simulink library "Library_Octocopter"  (R2015b)
settings: Solver=VariableStepAuto  StartTime=0.0  StopTime=10.0  RelTol=1e-3
values from neighbouring files (symbols this model uses):
  AoAMax = 18    [MainDataFile.m]
  ChordBlade = 0.2    [MainDataFile.m]
  DiameterBlade = 8    [MainDataFile.m]
  MassBlade = 35    [MainDataFile.m]
  RPMMax = 6400    [MainDataFile.m]
  s = saveObjectImpl@matlab.System(obj)    [moving_average.m]
  ThicknessBlade = 0.04    [MainDataFile.m]
  TransmissionRatio = 12    [MainDataFile.m]
undefined symbols (not defined in the file or in its folder): X, Y, Z
libraries: sm_lib x10, nesl_utility x9
settings Model: Creator=John  LastModifiedBy=hielke

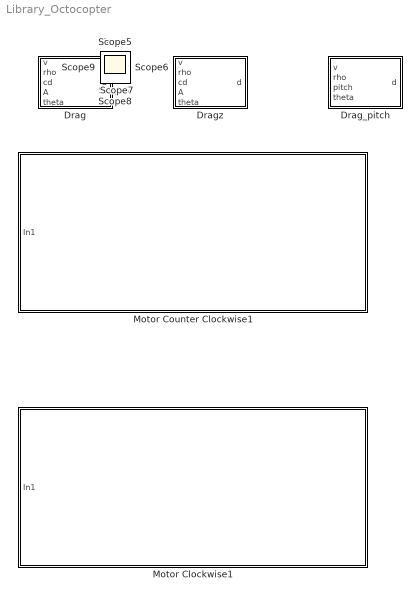
== system Library_Octocopter ==
  Drag : MATLAB Function  TreatAsAtomicUnit=on  SystemSampleTime=1
      settings: MinAlgLoopOccurrences=on  RTWSystemCode=Inline
  Drag_pitch : MATLAB Function  TreatAsAtomicUnit=on  SystemSampleTime=1
      settings: MinAlgLoopOccurrences=on  RTWSystemCode=Inline
  "Dragz " : MATLAB Function  TreatAsAtomicUnit=on  SystemSampleTime=1
      settings: MinAlgLoopOccurrences=on  RTWSystemCode=Inline
  Motor Clockwise1 : Subsystem
  Motor Counter Clockwise1 : Subsystem
  Scope{,1..9} (10 alike) : Scope

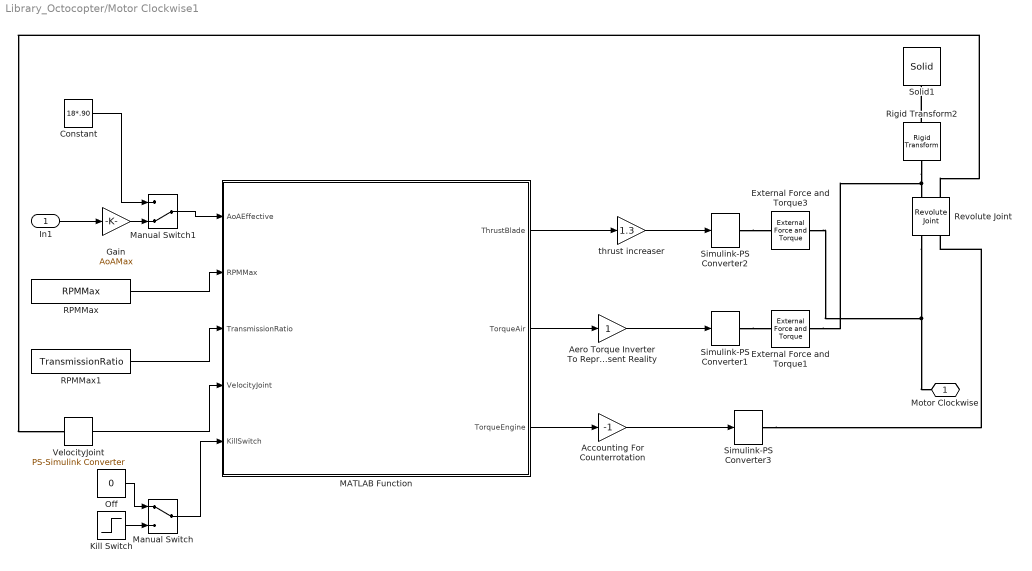
== system Library_Octocopter/Motor Clockwise1 ==
  In1 : Inport
  Accounting For Counterrotation : Gain  Gain=-1
  Aero Torque Inverter To Represent Reality : Gain
  Constant : Constant  Value=18*.90
  External Force and Torque1 : sm_lib/Forces and Torques/External Force and Torque  ForceResolutionFrame=AttachedFrame  EnableForceX=off  EnableForceY=off  EnableForceZ=off  EnableForce=off  TorqueResolutionFrame=AttachedFrame  EnableTorqueX=off  EnableTorqueY=off  EnableTorqueZ=on  EnableTorque=off  BlockFunction=simmechanics.library.forces_torques.external_force_torque
  External Force and Torque3 : sm_lib/Forces and Torques/External Force and Torque  ForceResolutionFrame=AttachedFrame  EnableForceX=off  EnableForceY=off  EnableForceZ=on  EnableForce=off  TorqueResolutionFrame=AttachedFrame  EnableTorqueX=off  EnableTorqueY=off  EnableTorqueZ=off  EnableTorque=off  BlockFunction=simmechanics.library.forces_torques.external_force_torque
  Gain : Gain  Gain=AoAMax
  Kill Switch : Step  Time=10
  MATLAB Function : MATLAB Function  TreatAsAtomicUnit=on
  Manual Switch : ManualSwitch
  Manual Switch1 : ManualSwitch  CurrentSetting=0
  Off : Constant  Value=0
  RPMMax : Constant  Value=RPMMax
  RPMMax1 : Constant  Value=TransmissionRatio
  Revolute Joint : sm_lib/Joints/Revolute Joint  SenseConstraintForce=off  SenseConstraintForceX=off  SenseConstraintForceY=off  SenseConstraintForceZ=off  SenseConstraintTorque=off  SenseConstraintTorqueX=off  SenseConstraintTorqueY=off  SenseConstraintTorqueZ=off  SenseTotalForce=off  SenseTotalForceX=off  SenseTotalForceY=off  SenseTotalForceZ=off  SenseTotalTorque=off  SenseTotalTorqueX=off  SenseTotalTorqueY=off  SenseTotalTorqueZ=off  CompositeWrenchDir=FollowerOnBase  CompositeWrenchFrame=BaseFrame  EquilibriumPosition=0  EquilibriumPositionUnits=deg  SpringStiffness=0  SpringStiffnessUnits=N*m/deg  DampingCoefficient=0  DampingCoefficientUnits=N*m/(deg/s)  TorqueActuationMode=InputTorque  MotionActuationMode=ComputedMotion  SensePosition=off  SenseVelocity=on  SenseAcceleration=off  SenseTorqueForce=off  PositionTargetSpecify=off  PositionTargetPriority=High  PositionTargetValue=0  PositionTargetValueUnits=deg  VelocityTargetSpecify=off  VelocityTargetPriority=High  VelocityTargetValue=0  VelocityTargetValueUnits=deg/s  BlockFunction=simmechanics.library.joints.revolute_joint
  Rigid Transform2 : sm_lib/Frames and Transforms/Rigid Transform  TranslationMethod=None  TranslationLengthUnit=m  TranslationStandardAxis=+Z  TranslationStandardOffset=0  TranslationCartesianOffset=[0 0 0]  TranslationROffset=0  TranslationROffsetUnits=m  TranslationZOffset=0  TranslationZOffsetUnits=m  TranslationThetaOffset=0  TranslationThetaOffsetUnits=deg  RotationMethod=StandardAxis  RotationAngleUnits=deg  RotationStandardAxis=+X  RotationAngle=90  RotationArbitraryAxis=[0 0 1]  FollAlignAxisA=+X  BaseAlignAxisA=+Y  FollAlignAxisB=+Y  BaseAlignAxisB=+Z  RotationSequenceAxes=FollowerAxes  RotationSequence=XYX  RotationSequenceAngles=[0 0 0]  RotationSequenceAnglesUnits=deg  RotationMatrix=[1 0 0; 0 1 0; 0 0 1]  BlockFunction=simmechanics.library.frames_transforms.rigid_transform
  Simulink-PS Converter1 : nesl_utility/Simulink-PS Converter  PhysicalDomain=network_engine_domain  SubClassName=ps_input  LeftPortType=input  RightPortType=output  PseudoPeriodic=off  Frequencies=[]  NoiseDistribution=none  NoiseParameters=[]  Unit=1  AffineConversion=off  InputFiltering=off  SimscapeFilterOrder=1  InputFilterTimeConstant=0.001  UdotUserProvided=1
  Simulink-PS Converter2 : nesl_utility/Simulink-PS Converter  PhysicalDomain=network_engine_domain  SubClassName=ps_input  LeftPortType=input  RightPortType=output  PseudoPeriodic=off  Frequencies=[]  NoiseDistribution=none  NoiseParameters=[]  Unit=1  AffineConversion=off  InputFiltering=off  SimscapeFilterOrder=1  InputFilterTimeConstant=0.001  UdotUserProvided=1
  Simulink-PS Converter3 : nesl_utility/Simulink-PS Converter  PhysicalDomain=network_engine_domain  SubClassName=ps_input  LeftPortType=input  RightPortType=output  PseudoPeriodic=off  Frequencies=[]  NoiseDistribution=none  NoiseParameters=[]  Unit=1  AffineConversion=off  InputFiltering=off  SimscapeFilterOrder=1  InputFilterTimeConstant=0.001  UdotUserProvided=1
  Solid1 : sm_lib/Body Elements/Solid  InertiaType=CalculateFromGeometry  Mass=MassBlade  MassUnits=kg  CenterOfMass=[0 0 0]  CenterOfMassUnits=m  MomentsOfInertia=[1 1 1]  MomentsOfInertiaUnits=kg*m^2  ProductsOfInertia=[0 0 0]  ProductsOfInertiaUnits=kg*m^2  DensityBased=off  Density=DensityBlade  DensityUnits=kg/(m^3)  DoExposeReferenceFrame=on  SerializedFrames=<Frames/>  GraphicType=FromGeometry  MarkerShape=Sphere  MarkerSize=10  MarkerSizeUnits=m  GraphicVisPropType=SimpleVisualProperties  GraphicDiffuseColor=[0.5 0.5 0.5]  GraphicSpecularColor=[0.5 0.5 0.5 1.0]  GraphicAmbientColor=[0.15 0.15 0.15 1.0]  GraphicEmissiveColor=[0.0 0.0 0.0 1.0]  GraphicShininess=75  GraphicOpacity=1.0  GeometryShape=Ellipsoid  RectangleSize=[1 1]  RectangleSizeUnits=m  BrickDimensions=[1 1 1]  BrickDimensionUnits=m  CylinderRadius=1  CylinderRadiusUnits=m  CylinderLength=1  CylinderLengthUnits=m  SphereRadius=1  SphereRadiusUnits=m  EllipsoidRadii=[DiameterBlade/2 ThicknessBlade/2 ChordBlade/2]  EllipsoidRadiiUnits=m  ExtrusionCrossSection=[1 1; -1 1; -1 -1; 1 -1]  ExtrusionCrossSectionUnits=m  ExtrusionLength=1  ExtrusionLengthUnits=m  PolygonNumSides=3  PolygonOuterRadius=1  PolygonOuterRadiusUnits=m  ExtGeomFileType=STL  ExtGeomFileName=Helice_Valor predeterminado_sldprt.STL  ExtGeomFileUnits=m  RevolutionCrossSection=[1 1; 1 -1; 2 -1; 2 1]  RevolutionCrossSectionUnits=m  RevolutionExtent=Full  RevolutionAngle=180  RevolutionAngleUnits=deg  BlockFunction=simmechanics.library.body_elements.solid
  VelocityJoint : nesl_utility/PS-Simulink Converter  PhysicalDomain=network_engine_domain  SubClassName=ps_output  LeftPortType=input  RightPortType=output  PseudoPeriodic=off  Frequencies=[]  Unit=1  AffineConversion=off
  thrust increaser : Gain  Gain=1.3
  Motor Clockwise : PMIOPort  Port=1  Side=Right
  wires:
  Accounting For Counterrotation/1 -> Simulink-PS Converter3/1
  MATLAB Function/1(ThrustBlade) -> thrust increaser/1
  In1/1 -> Gain/1
  RPMMax/1 -> MATLAB Function/2(RPMMax)
  RPMMax1/1 -> MATLAB Function/3(TransmissionRatio)
  MATLAB Function/2(TorqueAir) -> Aero Torque Inverter To Represent Reality/1
  Aero Torque Inverter To Represent Reality/1 -> Simulink-PS Converter1/1
  VelocityJoint/1 -> MATLAB Function/4(VelocityJoint)
  MATLAB Function/3(TorqueEngine) -> Accounting For Counterrotation/1
  Kill Switch/1 -> Manual Switch/2
  Off/1 -> Manual Switch/1
  Manual Switch/1 -> MATLAB Function/5(KillSwitch)
  Gain/1 -> Manual Switch1/2
  Manual Switch1/1 -> MATLAB Function/1(AoAEffective)
  Constant/1 -> Manual Switch1/1
  thrust increaser/1 -> Simulink-PS Converter2/1
  connections:
  Rigid Transform2/LConn1 -- Solid1/RConn1
  Rigid Transform2/RConn1 -- External Force and Torque1/RConn1 -- Revolute Joint/RConn1
  Revolute Joint/LConn1 -- Motor Clockwise/RConn1 -- External Force and Torque3/RConn1
  Simulink-PS Converter3/RConn1 -- Revolute Joint/LConn2
  Simulink-PS Converter2/RConn1 -- External Force and Torque3/LConn1
  Simulink-PS Converter1/RConn1 -- External Force and Torque1/LConn1
  Revolute Joint/RConn2 -- VelocityJoint/LConn1

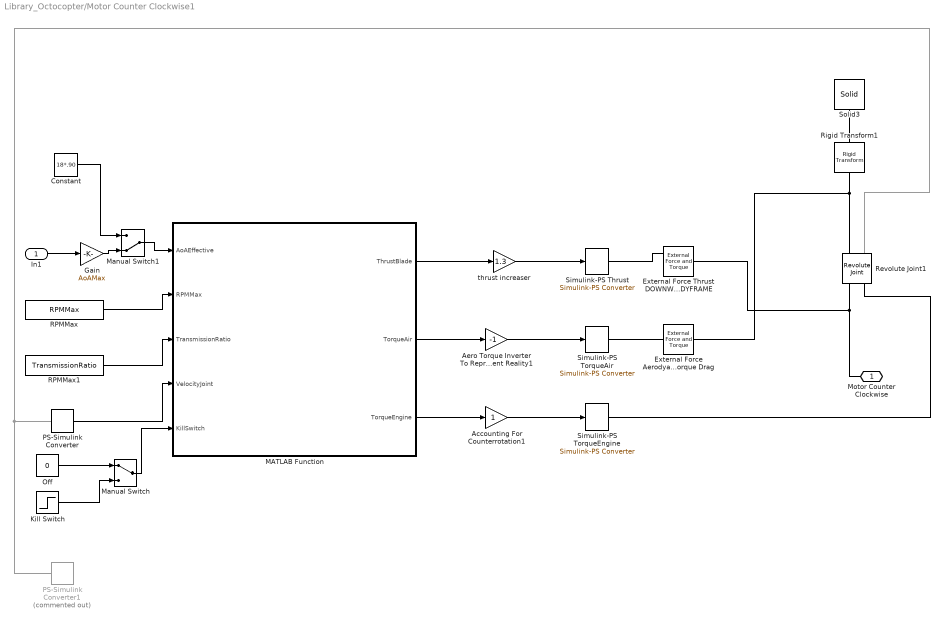
== system Library_Octocopter/Motor Counter Clockwise1 ==
  In1 : Inport
  Accounting For Counterrotation1 : Gain
  Aero Torque Inverter To Represent Reality1 : Gain  Gain=-1
  Constant : Constant  Value=18*.90
  External Force Aerodyanic Torque Drag : sm_lib/Forces and Torques/External Force and Torque  ForceResolutionFrame=AttachedFrame  EnableForceX=off  EnableForceY=off  EnableForceZ=off  EnableForce=off  TorqueResolutionFrame=AttachedFrame  EnableTorqueX=off  EnableTorqueY=off  EnableTorqueZ=on  EnableTorque=off  BlockFunction=simmechanics.library.forces_torques.external_force_torque
  External Force Thrust DOWNWARD Z BODYFRAME : sm_lib/Forces and Torques/External Force and Torque  ForceResolutionFrame=AttachedFrame  EnableForceX=off  EnableForceY=off  EnableForceZ=on  EnableForce=off  TorqueResolutionFrame=AttachedFrame  EnableTorqueX=off  EnableTorqueY=off  EnableTorqueZ=on  EnableTorque=off  BlockFunction=simmechanics.library.forces_torques.external_force_torque
  Gain : Gain  Gain=AoAMax
  Kill Switch : Step  Time=10
  MATLAB Function : MATLAB Function  TreatAsAtomicUnit=on
  Manual Switch : ManualSwitch
  Manual Switch1 : ManualSwitch  CurrentSetting=0
  Off : Constant  Value=0
  PS-Simulink Converter : nesl_utility/PS-Simulink Converter  PhysicalDomain=network_engine_domain  SubClassName=ps_output  LeftPortType=input  RightPortType=output  PseudoPeriodic=off  Frequencies=[]  Unit=1  AffineConversion=off
  PS-Simulink Converter1 : nesl_utility/PS-Simulink Converter  Commented=on  PhysicalDomain=network_engine_domain  SubClassName=ps_output  LeftPortType=input  RightPortType=output  PseudoPeriodic=off  Frequencies=[]  Unit=1  AffineConversion=off
  RPMMax : Constant  Value=RPMMax
  RPMMax1 : Constant  Value=TransmissionRatio
  Revolute Joint1 : sm_lib/Joints/Revolute Joint  SenseConstraintForce=off  SenseConstraintForceX=off  SenseConstraintForceY=off  SenseConstraintForceZ=off  SenseConstraintTorque=off  SenseConstraintTorqueX=off  SenseConstraintTorqueY=off  SenseConstraintTorqueZ=off  SenseTotalForce=off  SenseTotalForceX=off  SenseTotalForceY=off  SenseTotalForceZ=off  SenseTotalTorque=off  SenseTotalTorqueX=off  SenseTotalTorqueY=off  SenseTotalTorqueZ=off  CompositeWrenchDir=FollowerOnBase  CompositeWrenchFrame=BaseFrame  EquilibriumPosition=0  EquilibriumPositionUnits=deg  SpringStiffness=0  SpringStiffnessUnits=N*m/deg  DampingCoefficient=0  DampingCoefficientUnits=N*m/(deg/s)  TorqueActuationMode=InputTorque  MotionActuationMode=ComputedMotion  SensePosition=off  SenseVelocity=on  SenseAcceleration=off  SenseTorqueForce=off  PositionTargetSpecify=off  PositionTargetPriority=High  PositionTargetValue=0  PositionTargetValueUnits=deg  VelocityTargetSpecify=off  VelocityTargetPriority=High  VelocityTargetValue=0  VelocityTargetValueUnits=deg/s  BlockFunction=simmechanics.library.joints.revolute_joint
  Rigid Transform1 : sm_lib/Frames and Transforms/Rigid Transform  TranslationMethod=None  TranslationLengthUnit=m  TranslationStandardAxis=+Z  TranslationStandardOffset=0  TranslationCartesianOffset=[0 0 0]  TranslationROffset=0  TranslationROffsetUnits=m  TranslationZOffset=0  TranslationZOffsetUnits=m  TranslationThetaOffset=0  TranslationThetaOffsetUnits=deg  RotationMethod=StandardAxis  RotationAngleUnits=deg  RotationStandardAxis=+X  RotationAngle=90  RotationArbitraryAxis=[0 0 1]  FollAlignAxisA=+X  BaseAlignAxisA=+Y  FollAlignAxisB=+Y  BaseAlignAxisB=+Z  RotationSequenceAxes=FollowerAxes  RotationSequence=XYX  RotationSequenceAngles=[0 0 0]  RotationSequenceAnglesUnits=deg  RotationMatrix=[1 0 0; 0 1 0; 0 0 1]  BlockFunction=simmechanics.library.frames_transforms.rigid_transform
  Simulink-PS Thrust : nesl_utility/Simulink-PS Converter  PhysicalDomain=network_engine_domain  SubClassName=ps_input  LeftPortType=input  RightPortType=output  PseudoPeriodic=off  Frequencies=[]  NoiseDistribution=none  NoiseParameters=[]  Unit=1  AffineConversion=off  InputFiltering=off  SimscapeFilterOrder=1  InputFilterTimeConstant=0.001  UdotUserProvided=1
  Simulink-PS TorqueAir : nesl_utility/Simulink-PS Converter  PhysicalDomain=network_engine_domain  SubClassName=ps_input  LeftPortType=input  RightPortType=output  PseudoPeriodic=off  Frequencies=[]  NoiseDistribution=none  NoiseParameters=[]  Unit=1  AffineConversion=off  InputFiltering=off  SimscapeFilterOrder=1  InputFilterTimeConstant=0.001  UdotUserProvided=1
  Simulink-PS TorqueEngine : nesl_utility/Simulink-PS Converter  PhysicalDomain=network_engine_domain  SubClassName=ps_input  LeftPortType=input  RightPortType=output  PseudoPeriodic=off  Frequencies=[]  NoiseDistribution=none  NoiseParameters=[]  Unit=1  AffineConversion=off  InputFiltering=off  SimscapeFilterOrder=1  InputFilterTimeConstant=0.001  UdotUserProvided=1
  Solid3 : sm_lib/Body Elements/Solid  InertiaType=CalculateFromGeometry  Mass=MassBlade  MassUnits=kg  CenterOfMass=[0 0 0]  CenterOfMassUnits=m  MomentsOfInertia=[1 1 1]  MomentsOfInertiaUnits=kg*m^2  ProductsOfInertia=[0 0 0]  ProductsOfInertiaUnits=kg*m^2  DensityBased=off  Density=DensityBlade  DensityUnits=kg/(m^3)  DoExposeReferenceFrame=on  SerializedFrames=<Frames/>  GraphicType=FromGeometry  MarkerShape=Sphere  MarkerSize=10  MarkerSizeUnits=m  GraphicVisPropType=SimpleVisualProperties  GraphicDiffuseColor=[0.5 0.5 0.5]  GraphicSpecularColor=[0.5 0.5 0.5 1.0]  GraphicAmbientColor=[0.15 0.15 0.15 1.0]  GraphicEmissiveColor=[0.0 0.0 0.0 1.0]  GraphicShininess=75  GraphicOpacity=1.0  GeometryShape=Ellipsoid  RectangleSize=[1 1]  RectangleSizeUnits=m  BrickDimensions=[1 1 1]  BrickDimensionUnits=m  CylinderRadius=1  CylinderRadiusUnits=m  CylinderLength=1  CylinderLengthUnits=m  SphereRadius=1  SphereRadiusUnits=m  EllipsoidRadii=[DiameterBlade/2 ThicknessBlade/2 ChordBlade/2]  EllipsoidRadiiUnits=m  ExtrusionCrossSection=[1 1; -1 1; -1 -1; 1 -1]  ExtrusionCrossSectionUnits=m  ExtrusionLength=1  ExtrusionLengthUnits=m  PolygonNumSides=3  PolygonOuterRadius=1  PolygonOuterRadiusUnits=m  ExtGeomFileType=STL  ExtGeomFileName=Helice_Valor predeterminado_sldprt.STL  ExtGeomFileUnits=m  RevolutionCrossSection=[1 1; 1 -1; 2 -1; 2 1]  RevolutionCrossSectionUnits=m  RevolutionExtent=Full  RevolutionAngle=180  RevolutionAngleUnits=deg  BlockFunction=simmechanics.library.body_elements.solid
  thrust increaser : Gain  Gain=1.3
  Motor Counter Clockwise : PMIOPort  Port=1  Side=Right
  wires:
  In1/1 -> Gain/1
  MATLAB Function/1(ThrustBlade) -> thrust increaser/1
  RPMMax/1 -> MATLAB Function/2(RPMMax)
  RPMMax1/1 -> MATLAB Function/3(TransmissionRatio)
  PS-Simulink Converter/1 -> MATLAB Function/4(VelocityJoint)
  Off/1 -> Manual Switch/1
  Manual Switch/1 -> MATLAB Function/5(KillSwitch)
  Kill Switch/1 -> Manual Switch/2
  MATLAB Function/2(TorqueAir) -> Aero Torque Inverter To Represent Reality1/1
  MATLAB Function/3(TorqueEngine) -> Accounting For Counterrotation1/1
  Aero Torque Inverter To Represent Reality1/1 -> Simulink-PS TorqueAir/1
  Accounting For Counterrotation1/1 -> Simulink-PS TorqueEngine/1
  Constant/1 -> Manual Switch1/1
  Manual Switch1/1 -> MATLAB Function/1(AoAEffective)
  Gain/1 -> Manual Switch1/2
  thrust increaser/1 -> Simulink-PS Thrust/1
  connections:
  PS-Simulink Converter1/LConn1 -- Revolute Joint1/RConn2 -- PS-Simulink Converter/LConn1
  Revolute Joint1/LConn1 -- Motor Counter Clockwise/RConn1 -- External Force Thrust DOWNWARD Z BODYFRAME/RConn1
  Simulink-PS Thrust/RConn1 -- External Force Thrust DOWNWARD Z BODYFRAME/LConn1
  External Force Aerodyanic Torque Drag/LConn1 -- Simulink-PS TorqueAir/RConn1
  Simulink-PS TorqueEngine/RConn1 -- Revolute Joint1/LConn2
  Revolute Joint1/RConn1 -- Rigid Transform1/LConn1 -- External Force Aerodyanic Torque Drag/RConn1
  Rigid Transform1/RConn1 -- Solid3/RConn1

== matlab function Library_Octocopter/Motor Counter Clockwise1/MATLAB Function ==
  data: AoAEffective input; RPMMax input; TransmissionRatio input; ThrustBlade output; TorqueAir output; TorqueEngine output; VelocityJoint input; KillSwitch input
function [ThrustBlade,TorqueAir, TorqueEngine] = AeroThrustTorque2(AoAEffective, RPMMax, TransmissionRatio, VelocityJoint, KillSwitch)

%%%Compute the rotational velocity after transmission in rad/s%%%
RPMMaxtoRadafterTransmission=(RPMMax*(pi/30))/TransmissionRatio;

%%%Round the pitch setting to one decimal (x.x)%%%
AoAEffectiveRound=round(AoAEffective*10);

%%%The Pitch Blade setting is chosen form 181 options (18 degree with 0.1
%%%increment); +1 is used since the first data point is 0 degrees pitch%%%
AoAEffectiveIndex=AoAEffectiveRound+1;

%%%Thrust/Torque vector values for each pitch setting from 0.0 to 18.0, independent of angular velocity%%%
ThrustVector=[541.847560609448;896.118838323176;2151.76915659467;1216.88036795354;1064.48391982187;1051.28460160294;1089.35830550795;1152.17008024410;1228.30130123324;1312.12403081697;1400.66604764224;1492.28957524919;1586.06407446818;1681.44710303351;1778.11452516211;1875.86732238593;1974.57924966392;2074.16690453835;2174.57237174159;2275.75305039650;2377.67564327290;2480.31258600908;2583.63991980096;2687.63602371813;2792.28086104767;2897.55553340609;3003.44201876345;3109.92301871547;3216.98186993036;3324.60249260364;3432.76935963347;3541.46747685132;3650.68236867222;3760.40006597063;3870.60709445643;3981.29046269727;4092.43764943873;4204.03659015676;4316.07566292560;4428.54367375305;4541.42984155795;4654.72378296186;4768.41549705123;4882.49535024486;4996.95406137822;5111.78268709429;5226.97260761029;5342.51551291215;5458.40338941356;5574.62850710396;5691.18340719957;5808.06089030325;5925.25400507247;6042.75603738951;6160.56050002413;6278.66112277581;6397.05184308079;6515.72679706742;6634.68031104245;6753.90689339040;6873.40122686779;6993.15816127412;7113.17270648180;7233.44002580739;7353.95542970724;7474.71436978099;7595.71243306717;7716.94533661564;7838.40892232237;7960.09915201280;8082.01210276043;8204.14396242837;8326.49102542177;8449.04968864005;8571.81644761818;8694.78789284708;8817.96070626358;8941.33165790090;9064.89760269133;9188.65547741306;9312.60229777353;9436.73515562241;9561.05121628720;9685.54771602546;9810.22195958742;9935.07131788353;10060.0932257515;10185.2851798181;10310.6447364502;10436.1695097923;10561.8571698838;10687.7054408545;10813.7120991933;10939.8749720861;11066.1919358216;11192.6609142585;11319.2798773552;11446.0468397552;11572.9598594281;11700.0170363635;11827.2165113130;11954.5564645819;12082.0351148648;12209.6507181252;12337.4015665164;12465.2859873422;12593.3023420553;12721.4490252920;12849.7244639411;12978.1271162469;13106.6554709427;13235.3080464158;13364.0833899008;13492.9800767011;13621.9967094370;13751.1319173197;13880.3843554492;14009.7527041365;14139.2356682478;14268.8319765709;14398.5403812020;14528.3596569526;14658.2886007757;14788.3260312105;14918.4707878447;15048.7217307940;15179.0777401978;15309.5377157306;15440.1005761292;15570.7652587339;15701.5307190437;15832.3959302856;15963.3598829965;16094.4215846176;16225.5800591014;16356.8343465298;16488.1835027441;16619.6265989847;16751.1627215429;16882.7909714213;17014.5104640047;17146.3203287406;17278.2197088277;17410.2077609146;17542.2836548060;17674.4465731773;17806.6957112971;17939.0302767574;18071.4494892112;18203.9525801173;18336.5387924915;18469.2073806653;18601.9576100505;18734.7887569099;18867.7001081346;19000.6909610267;19133.7606230881;19266.9084118141;19400.1336544931;19533.4356880108;19666.8138586599;19800.2675219542;19933.7960424478;20067.3987935584;20201.0751573952;20334.8245245915;20468.6462941405;20602.5398732360;20736.5046771165;20870.5401289133;21004.6456595022;21138.8207073586;21273.0647184164;21407.3771459301;21541.7574503399;21676.2050991404;21810.7195667522;21945.3003343962;22079.9468899716;22214.6587279355;22349.4353491865];
TorqueVector=[1459.51361152833;1476.96071665212;1477.24976063132;1434.28211646647;1421.21221602182;1416.26545740138;1415.19692220516;1416.34208800097;1418.88959831949;1422.41225194972;1426.67580746483;1431.54802999146;1436.95225586016;1442.84273789966;1449.19121025913;1455.97942262001;1463.19492625960;1470.82866538491;1478.87358664918;1487.32383064858;1496.17425977511;1505.42018217952;1515.05719079766;1525.08107012649;1535.48774290079;1546.27324017893;1557.43368503506;1568.96528402657;1580.86432297744;1593.12716503978;1605.75024985062;1618.73009311295;1632.06328623581;1645.74649584918;1659.77646311414;1674.15000280773;1688.86400219406;1703.91541970822;1719.30128348580;1735.01868977141;1751.06480123754;1767.43684524173;1784.13211204610;1801.14795301937;1818.48177883814;1836.13105770087;1854.09331356508;1872.36612441634;1890.94712057516;1909.83398304654;1929.02444191558;1948.51627479128;1968.30730529989;1988.39540162845;2008.77847511856;2029.45447891008;2050.42140663382;2071.67729115252;2093.22020334864;2115.04825095791;2137.15957744697;2159.55236093380;2182.22481314934;2205.17517843870;2228.40173280062;2251.90278296344;2275.67666549627;2299.72174595378;2324.03641805335;2348.61910288300;2373.46824813900;2398.58232739180;2423.95983937895;2449.59930732410;2475.49927828062;2501.65832249914;2528.07503281766;2554.74802407342;2581.67593253560;2608.85741535787;2636.29115005002;2663.97583396782;2691.91018382036;2720.09293519411;2748.52284209297;2777.19867649381;2806.11922791659;2835.28330300871;2864.68972514283;2894.33733402775;2924.22498533170;2954.35155031768;2984.71591549018;3015.31698225307;3046.15366657800;3077.22489868302;3108.52962272103;3140.06679647766;3171.83539107811;3203.83439070286;3236.06279231166;3268.51960537567;3301.20385161735;3334.11456475784;3367.25079027159;3400.61158514790;3434.19601765926;3468.00316713609;3502.03212374769;3536.28198828933;3570.75187197505;3605.44089623611;3640.34819252487;3675.47290212385;3710.81417595991;3746.37117442328;3782.14306719134;3818.12903305690;3854.32825976096;3890.73994382974;3927.36329041579;3964.19751314313;4001.24183395629;4038.49548297300;4075.95769834065;4113.62772609613;4151.50482002914;4189.58824154882;4227.87725955350;4266.37115030364;4305.06919729770;4343.97069115098;4383.07492947724;4422.38121677314;4461.88886430519;4501.59718999952;4541.50551833389;4581.61318023236;4621.91951296219;4662.42386003309;4703.12557109869;4744.02400186021;4785.11851397215;4826.40847495015;4867.89325808076;4909.57224233315;4951.44481227273;4993.51035797664;5035.76827495089;5078.21796404940;5120.85883139463;5163.69028829985;5206.71175119305;5249.92264154240;5293.32238578321;5336.91041524638;5380.68616608828;5424.64907922203;5468.79860025018;5513.13417939866;5557.65527145211;5602.36133569037;5647.25183582631;5692.32623994480;5737.58402044285;5783.02465397095;5828.64762137545;5874.45240764208;5920.43850184055;5966.60539707010;6012.95259040619;6059.47958284804;6106.18587926724;6153.07098835726;6200.13442258390;6247.37569813657;6294.79433488057;6342.38985631011;6390.16178950224;6438.10966507155;6486.23301712573];

%%%Compute the torque the engine can deliver as a function of rotational
%%%velocity%%%
if KillSwitch == 0 && abs(VelocityJoint) >= 0 && abs(VelocityJoint) < 34.9
TorqueProvided=((abs(VelocityJoint)*(30*TransmissionRatio/pi)-1000)*0.119615+570)*TransmissionRatio;
elseif KillSwitch == 0 && abs(VelocityJoint) >= 34.9 && abs(VelocityJoint) <56.7
TorqueProvided=((abs(VelocityJoint)*(30*TransmissionRatio/pi)-3600)*-0.05821+881)*TransmissionRatio;
elseif KillSwitch == 0 && abs(VelocityJoint) >= 56.8
TorqueProvided=0;
else
TorqueProvided = 0;
end

%%%Max angular velocity engine - actual velocity blade%%
%%%NOTE: If VelocityNet=<0, the blade has reached max angular velocity and
%%%is limited by the engine%%%
VelocityNet=RPMMaxtoRadafterTransmission-abs(VelocityJoint);

%%%Torque from air on body (rotor?)%%%
if KillSwitch == 0 && VelocityNet>55
TorqueAir=0;
elseif KillSwitch == 0 && VelocityNet<=45
TorqueAir=TorqueVector(AoAEffectiveIndex);
else
TorqueAir=TorqueVector(AoAEffectiveIndex)*(abs(VelocityJoint)/RPMMaxtoRadafterTransmission);
end



if KillSwitch == 0 && VelocityNet > 0
    ThrustBlade = ThrustVector(AoAEffectiveIndex);
    TorqueEngine = TorqueProvided;
elseif KillSwitch == 0 && VelocityNet <= 0
    ThrustBlade = ThrustVector(AoAEffectiveIndex);
    TorqueEngine = TorqueVector(AoAEffectiveIndex);
elseif KillSwitch == 1 && abs(VelocityJoint) > 0
    ThrustBlade = ThrustVector(AoAEffectiveIndex)*(abs(VelocityJoint)/RPMMaxtoRadafterTransmission);
    TorqueEngine = TorqueProvided;
else
    ThrustBlade =0;
    TorqueEngine =0;
end
end

== matlab function Library_Octocopter/Motor Clockwise1/MATLAB Function ==
  data: AoAEffective input; RPMMax input; TransmissionRatio input; ThrustBlade output; TorqueAir output; TorqueEngine output; VelocityJoint input; KillSwitch input
function [ThrustBlade,TorqueAir, TorqueEngine] = AeroThrustTorque2(AoAEffective, RPMMax, TransmissionRatio, VelocityJoint, KillSwitch)

%%%Compute the rotational velocity after transmission in rad/s%%%
RPMMaxtoRadafterTransmission=(RPMMax*(pi/30))/TransmissionRatio;

%%%Round the pitch setting to one decimal (x.x)%%%
AoAEffectiveRound=round(AoAEffective*10);

%%%The Pitch Blade setting is chosen form 181 options (18 degree with 0.1
%%%increment); +1 is used since the first data point is 0 degrees pitch%%%
AoAEffectiveIndex=AoAEffectiveRound+1;

%%%Thrust/Torque vector values for each pitch setting from 0.0 to 18.0, independent of angular velocity%%%
ThrustVector=[541.847560609448;896.118838323176;2151.76915659467;1216.88036795354;1064.48391982187;1051.28460160294;1089.35830550795;1152.17008024410;1228.30130123324;1312.12403081697;1400.66604764224;1492.28957524919;1586.06407446818;1681.44710303351;1778.11452516211;1875.86732238593;1974.57924966392;2074.16690453835;2174.57237174159;2275.75305039650;2377.67564327290;2480.31258600908;2583.63991980096;2687.63602371813;2792.28086104767;2897.55553340609;3003.44201876345;3109.92301871547;3216.98186993036;3324.60249260364;3432.76935963347;3541.46747685132;3650.68236867222;3760.40006597063;3870.60709445643;3981.29046269727;4092.43764943873;4204.03659015676;4316.07566292560;4428.54367375305;4541.42984155795;4654.72378296186;4768.41549705123;4882.49535024486;4996.95406137822;5111.78268709429;5226.97260761029;5342.51551291215;5458.40338941356;5574.62850710396;5691.18340719957;5808.06089030325;5925.25400507247;6042.75603738951;6160.56050002413;6278.66112277581;6397.05184308079;6515.72679706742;6634.68031104245;6753.90689339040;6873.40122686779;6993.15816127412;7113.17270648180;7233.44002580739;7353.95542970724;7474.71436978099;7595.71243306717;7716.94533661564;7838.40892232237;7960.09915201280;8082.01210276043;8204.14396242837;8326.49102542177;8449.04968864005;8571.81644761818;8694.78789284708;8817.96070626358;8941.33165790090;9064.89760269133;9188.65547741306;9312.60229777353;9436.73515562241;9561.05121628720;9685.54771602546;9810.22195958742;9935.07131788353;10060.0932257515;10185.2851798181;10310.6447364502;10436.1695097923;10561.8571698838;10687.7054408545;10813.7120991933;10939.8749720861;11066.1919358216;11192.6609142585;11319.2798773552;11446.0468397552;11572.9598594281;11700.0170363635;11827.2165113130;11954.5564645819;12082.0351148648;12209.6507181252;12337.4015665164;12465.2859873422;12593.3023420553;12721.4490252920;12849.7244639411;12978.1271162469;13106.6554709427;13235.3080464158;13364.0833899008;13492.9800767011;13621.9967094370;13751.1319173197;13880.3843554492;14009.7527041365;14139.2356682478;14268.8319765709;14398.5403812020;14528.3596569526;14658.2886007757;14788.3260312105;14918.4707878447;15048.7217307940;15179.0777401978;15309.5377157306;15440.1005761292;15570.7652587339;15701.5307190437;15832.3959302856;15963.3598829965;16094.4215846176;16225.5800591014;16356.8343465298;16488.1835027441;16619.6265989847;16751.1627215429;16882.7909714213;17014.5104640047;17146.3203287406;17278.2197088277;17410.2077609146;17542.2836548060;17674.4465731773;17806.6957112971;17939.0302767574;18071.4494892112;18203.9525801173;18336.5387924915;18469.2073806653;18601.9576100505;18734.7887569099;18867.7001081346;19000.6909610267;19133.7606230881;19266.9084118141;19400.1336544931;19533.4356880108;19666.8138586599;19800.2675219542;19933.7960424478;20067.3987935584;20201.0751573952;20334.8245245915;20468.6462941405;20602.5398732360;20736.5046771165;20870.5401289133;21004.6456595022;21138.8207073586;21273.0647184164;21407.3771459301;21541.7574503399;21676.2050991404;21810.7195667522;21945.3003343962;22079.9468899716;22214.6587279355;22349.4353491865];
TorqueVector=[1459.51361152833;1476.96071665212;1477.24976063132;1434.28211646647;1421.21221602182;1416.26545740138;1415.19692220516;1416.34208800097;1418.88959831949;1422.41225194972;1426.67580746483;1431.54802999146;1436.95225586016;1442.84273789966;1449.19121025913;1455.97942262001;1463.19492625960;1470.82866538491;1478.87358664918;1487.32383064858;1496.17425977511;1505.42018217952;1515.05719079766;1525.08107012649;1535.48774290079;1546.27324017893;1557.43368503506;1568.96528402657;1580.86432297744;1593.12716503978;1605.75024985062;1618.73009311295;1632.06328623581;1645.74649584918;1659.77646311414;1674.15000280773;1688.86400219406;1703.91541970822;1719.30128348580;1735.01868977141;1751.06480123754;1767.43684524173;1784.13211204610;1801.14795301937;1818.48177883814;1836.13105770087;1854.09331356508;1872.36612441634;1890.94712057516;1909.83398304654;1929.02444191558;1948.51627479128;1968.30730529989;1988.39540162845;2008.77847511856;2029.45447891008;2050.42140663382;2071.67729115252;2093.22020334864;2115.04825095791;2137.15957744697;2159.55236093380;2182.22481314934;2205.17517843870;2228.40173280062;2251.90278296344;2275.67666549627;2299.72174595378;2324.03641805335;2348.61910288300;2373.46824813900;2398.58232739180;2423.95983937895;2449.59930732410;2475.49927828062;2501.65832249914;2528.07503281766;2554.74802407342;2581.67593253560;2608.85741535787;2636.29115005002;2663.97583396782;2691.91018382036;2720.09293519411;2748.52284209297;2777.19867649381;2806.11922791659;2835.28330300871;2864.68972514283;2894.33733402775;2924.22498533170;2954.35155031768;2984.71591549018;3015.31698225307;3046.15366657800;3077.22489868302;3108.52962272103;3140.06679647766;3171.83539107811;3203.83439070286;3236.06279231166;3268.51960537567;3301.20385161735;3334.11456475784;3367.25079027159;3400.61158514790;3434.19601765926;3468.00316713609;3502.03212374769;3536.28198828933;3570.75187197505;3605.44089623611;3640.34819252487;3675.47290212385;3710.81417595991;3746.37117442328;3782.14306719134;3818.12903305690;3854.32825976096;3890.73994382974;3927.36329041579;3964.19751314313;4001.24183395629;4038.49548297300;4075.95769834065;4113.62772609613;4151.50482002914;4189.58824154882;4227.87725955350;4266.37115030364;4305.06919729770;4343.97069115098;4383.07492947724;4422.38121677314;4461.88886430519;4501.59718999952;4541.50551833389;4581.61318023236;4621.91951296219;4662.42386003309;4703.12557109869;4744.02400186021;4785.11851397215;4826.40847495015;4867.89325808076;4909.57224233315;4951.44481227273;4993.51035797664;5035.76827495089;5078.21796404940;5120.85883139463;5163.69028829985;5206.71175119305;5249.92264154240;5293.32238578321;5336.91041524638;5380.68616608828;5424.64907922203;5468.79860025018;5513.13417939866;5557.65527145211;5602.36133569037;5647.25183582631;5692.32623994480;5737.58402044285;5783.02465397095;5828.64762137545;5874.45240764208;5920.43850184055;5966.60539707010;6012.95259040619;6059.47958284804;6106.18587926724;6153.07098835726;6200.13442258390;6247.37569813657;6294.79433488057;6342.38985631011;6390.16178950224;6438.10966507155;6486.23301712573];

%%%Compute the torque the engine can deliver as a function of rotational
%%%velocity%%%
if KillSwitch == 0 && abs(VelocityJoint) >= 0 && abs(VelocityJoint) < 34.9
TorqueProvided=((abs(VelocityJoint)*(30*TransmissionRatio/pi)-1000)*0.119615+570)*TransmissionRatio;
elseif KillSwitch == 0 && abs(VelocityJoint) >= 34.9 && abs(VelocityJoint) <56.7
TorqueProvided=((abs(VelocityJoint)*(30*TransmissionRatio/pi)-3600)*-0.05821+881)*TransmissionRatio;
elseif KillSwitch == 0 && abs(VelocityJoint) >= 56.8
TorqueProvided=0;
else
TorqueProvided = 0;
end

%%%Max angular velocity engine - actual velocity blade%%
%%%NOTE: If VelocityNet=<0, the blade has reached max angular velocity and
%%%is limited by the engine%%%
VelocityNet=RPMMaxtoRadafterTransmission-abs(VelocityJoint);

%%%Torque from air on body (rotor?)%%%
if KillSwitch == 0 && VelocityNet>55
TorqueAir=0;
elseif KillSwitch == 0 && VelocityNet<=45
TorqueAir=TorqueVector(AoAEffectiveIndex);
else
TorqueAir=TorqueVector(AoAEffectiveIndex)*(abs(VelocityJoint)/RPMMaxtoRadafterTransmission);
end



if KillSwitch == 0 && VelocityNet > 0
    ThrustBlade = ThrustVector(AoAEffectiveIndex);
    TorqueEngine = TorqueProvided;
elseif KillSwitch == 0 && VelocityNet <= 0
    ThrustBlade = ThrustVector(AoAEffectiveIndex);
    TorqueEngine = TorqueVector(AoAEffectiveIndex);
elseif KillSwitch == 1 && abs(VelocityJoint) > 0
    ThrustBlade = ThrustVector(AoAEffectiveIndex)*(abs(VelocityJoint)/RPMMaxtoRadafterTransmission);
    TorqueEngine = TorqueProvided;
else
    ThrustBlade =0;
    TorqueEngine =0;
end
end

== matlab function Library_Octocopter/Drag_pitch ==
  data: v input; d output; rho input; pitch input; theta input
function d = fcn(v, rho, pitch, theta)
%#codegen

d = -double(pitch)*double(rho)*double(v)*(0.7-double(theta)*0.075);

== matlab function Library_Octocopter/Dragz  ==
  data: v input; d output; rho input; cd input; A input; theta input
function d = fcn(v, rho, cd, A, theta)
%#codegen

d = -0.5* rho* abs(v)*v*cd*A*(1+cos(theta));

== matlab function Library_Octocopter/Drag ==
  data: v input; d output; rho input; cd input; A input; theta input
function d = fcn(v, rho, cd, A, theta)
%#codegen

d = -0.5* rho* abs(v)*v*cd*A*(1+sin(theta));
